simulink model "openckttestsinglephasexmer"  (R2024b)
settings: Solver=ode23tb  StartTime=0.0  StopTime=5  MaxStep=1e-4  RelTol=1e-3
libraries: spsRMSLib x2, spsACVoltageSourceLib x1, spsCurrentMeasurementLib x1, spsLinearTransformerLib x1, spsPowerLib x1, spsVoltageMeasurementLib x1, sps_lib x1
settings Model: Creator=brain  LastModifiedBy=brain

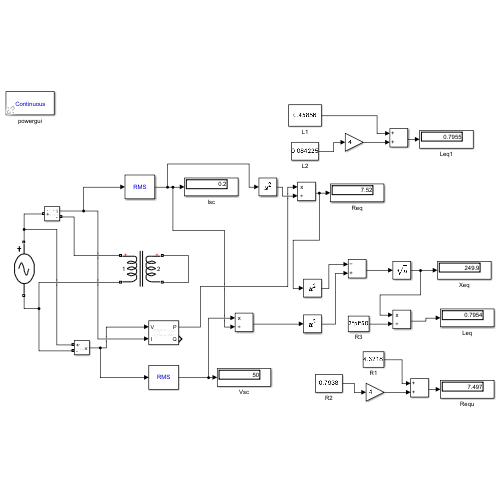
[thumbnail: Simulink's stored preview of the top-level diagram]
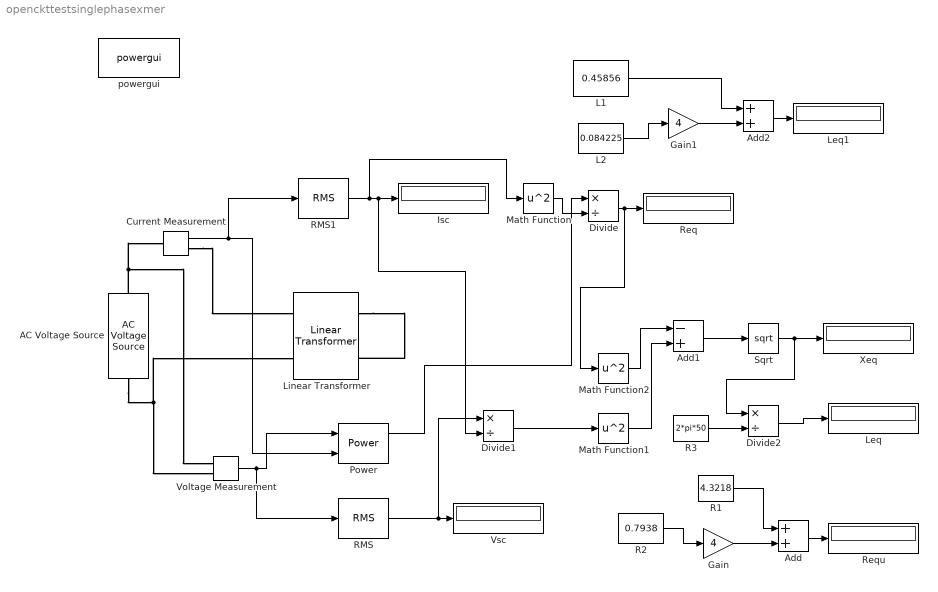
== system openckttestsinglephasexmer ==
  AC Voltage Source : spsACVoltageSourceLib/AC Voltage Source  Amplitude=50*sqrt(2)  Phase=0  Frequency=50  SampleTime=0  Measurements=None  BusType=swing  Pref=10e3  Qref=0  Qmin=-inf  Qmax=+inf
  Add : Sum
  Add1 : Sum  Inputs=-+
  Add2 : Sum
  Current Measurement : spsCurrentMeasurementLib/Current Measurement  PhasorSimulation=off  OutputType=Complex  PSBequivalent=0
  Divide : Product  Inputs=*/
  Divide1 : Product  Inputs=*/
  Divide2 : Product  Inputs=*/
  Gain : Gain  Gain=4
  Gain1 : Gain  Gain=4
  Isc : Display
  L1 : Constant  Value=0.45856
  L2 : Constant  Value=0.084225
  Leq : Display
  Leq1 : Display
  Linear Transformer : spsLinearTransformerLib/Linear Transformer  UNITS=SI  NominalPower=[2000 60 ]  winding1=[220 4.3218 0.45856]  winding2=[110 0.7938 0.084225]  ThreeWindings=off  winding3=[3.15e+05 0.7938 0.084225]  RmLm=[1.0804e+06 2866]  Measurements=None  DataType=on
  Math Function : Math  Operator=square
  Math Function1 : Math  Operator=square
  Math Function2 : Math  Operator=square
  Power : spsPowerLib/Power  Freq=50  Vinit=[1, 0]  Iinit=[1, 0]  Ts=0
  R1 : Constant  Value=4.3218
  R2 : Constant  Value=0.7938
  R3 : Constant  Value=2*pi*50
  RMS : spsRMSLib/RMS  TrueRMS=off  Freq=50  RMSInit=0  Ts=0
  RMS1 : spsRMSLib/RMS  TrueRMS=on  Freq=50  RMSInit=0  Ts=0
  Req : Display
  Requ : Display
  Sqrt : Sqrt
  Voltage Measurement : spsVoltageMeasurementLib/Voltage Measurement  PhasorSimulation=off  OutputType=Complex  PSBequivalent=0
  Vsc : Display
  Xeq : Display
  powergui : sps_lib/powergui  Priority=1  SimulationMode=Continuous  SampleTime=50e-6  frequency=60  Iterations=50  frequencyindice=50  Pbase=100e6  ErrMax=1e-4  UnitsV=kV  UnitsW=MW  buscounter=0  FunctionMessages=off  echomessages=off  EnableUseOfTLC=off  CurrentSourceSwitches=off  DisableSnubberDevices=off  DisableRonSwitches=off  DisableVfSwitches=off  DisplayEquations=off  AutomaticDiscreteSolvers=off  SolverType=Tustin/Backward Euler (TBE)  Interpol=off  ExternalGateDelay=off  methode=off  Ts=100  x0status=blocks  SPID=on  SwTol=0  HookPort=off  NonlinearTolerance=1e-4  nMaxIteration=100  ContinueOnMaxIteration=off  RestoreLinks=warning  ResistiveCurrentMeasurement=off  Frange=[0:2:500]  Ylog=off  Xlog=on  ShowGrid=off  save=off  variable=ZData  structure=0  ZoomFFT=off  StartTime=0.0  cycles=1  DisplayStyle=1  fundamental=60  FreqAxis=off  MaxFrequency=1000  frequencyindicesteady=1  RmsSteady=1  display=off
  wires:
  Current Measurement/1 -> RMS1/1, Power/2
  Voltage Measurement/1 -> RMS/1, Power/1
  RMS1/1 -> Divide1/2, Isc/1, Math Function/1
  RMS/1 -> Divide1/1, Vsc/1
  Power/1 -> Divide/1
  Math Function/1 -> Divide/2
  Divide/1 -> Math Function2/1, Req/1
  R2/1 -> Gain/1
  R1/1 -> Add/1
  Gain/1 -> Add/2
  Add/1 -> Requ/1
  Divide1/1 -> Math Function1/1
  Math Function1/1 -> Add1/2
  Math Function2/1 -> Add1/1
  Add1/1 -> Sqrt/1
  Sqrt/1 -> Divide2/1, Xeq/1
  R3/1 -> Divide2/2
  Divide2/1 -> Leq/1
  Add2/1 -> Leq1/1
  Gain1/1 -> Add2/2
  L1/1 -> Add2/1
  L2/1 -> Gain1/1
  connections:
  AC Voltage Source/LConn1 -- Voltage Measurement/LConn2 -- Linear Transformer/LConn2
  AC Voltage Source/RConn1 -- Voltage Measurement/LConn1 -- Current Measurement/LConn1
  Current Measurement/RConn1 -- Linear Transformer/LConn1
  Linear Transformer/RConn1 -- Linear Transformer/RConn2
